simulink model "full"  (Simulink 8.3)
settings: Solver=ode3  StartTime=0.0  StopTime=stop_time  FixedStep=step  RelTol=1e-3
values from neighbouring files (symbols this model uses):
  i_p = i_p_data(i)    [test_2.m]
  J_sum = J_d + 0.2*J_d + J_m/i_p^2    (= 0.011)    [test_2.m]
  K_a = 10/alpha_max    (= 1.5888147442)    [test_2.m]
  k_d = 1/R    (= 3.33333333333)    [test_2.m]
  k_e = U_n/w_0    (= 0.400454372941)    [test_2.m]
  K_I = 10/I_max    (= 0.108225108225)    [test_2.m]
  k_m = M_n/I_n    (= 0.400555555556)    [test_2.m]
  K_u = 10/U_n    (= 0.192307692308)    [test_2.m]
  K_w = 10/w_0    (= 0.0770104563348)    [test_2.m]
  k_y = U_n/U_m    (= 5.2)    [test_2.m]
  M_cm = 0    [test_2.m]
  T_y = 10*10^(-3)    (= 0.01)    [test_2.m]
  T_ya = 10*10^(-3)    (= 0.01)    [test_2.m]
  U = 5    [test_2.m]
settings Model: Creator=Павел  LastModifiedBy=Павел
settings DataIOCC: SignalLoggingSaveFormat=Dataset
settings DebuggingCC: UnderspecifiedInitializationDetection=Simplified  StateNameClashWarn=none
settings GRTTargetCC: CombineOutputUpdateFcns=on  GRTInterface=off

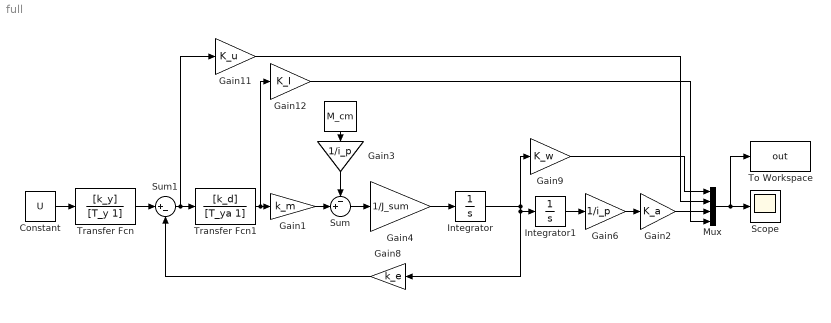
== system full ==
  " " : Constant  Value=M_cm
  Constant : Constant  Value=U
  Gain1 : Gain  Gain=k_m
  Gain11 : Gain  Gain=K_u
  Gain12 : Gain  Gain=K_I
  Gain2 : Gain  Gain=K_a
  Gain3 : Gain  Gain=1/i_p
  Gain4 : Gain  Gain=1/J_sum
  Gain6 : Gain  Gain=1/i_p
  Gain8 : Gain  Gain=k_e
  Gain9 : Gain  Gain=K_w
  Integrator : Integrator
  Integrator1 : Integrator
  Mux : Mux
  Scope : Scope
      settings: TimeRange=0.025712143928036  YMin=0.7292025862068964  YMax=0.7738146551724137
  Sum : Sum  Inputs=-+|
  Sum1 : Sum  Inputs=|+-
  To Workspace : ToWorkspace  VariableName=out  SaveFormat=Structure With Time  SampleTime=-1
  Transfer Fcn : TransferFcn  Numerator=[k_y]  Denominator=[T_y 1]
  Transfer Fcn1 : TransferFcn  Numerator=[k_d]  Denominator=[T_ya 1]
  wires:
  Sum1/1 -> Gain11/1, Transfer Fcn1/1
  Transfer Fcn/1 -> Sum1/1
  Constant/1 -> Transfer Fcn/1
  Gain1/1 -> Sum/2
  Gain3/1 -> Sum/1
  Sum/1 -> Gain4/1
  Gain4/1 -> Integrator/1
  Integrator/1 -> Gain9/1, Integrator1/1, Gain8/1
  Gain8/1 -> Sum1/2
  " "/1 -> Gain3/1
  Mux/1 -> Scope/1, To Workspace/1
  Transfer Fcn1/1 -> Gain12/1, Gain1/1
  Gain9/1 -> Mux/1
  Gain2/1 -> Mux/3
  Gain6/1 -> Gain2/1
  Integrator1/1 -> Gain6/1
  Gain11/1 -> Mux/2
  Gain12/1 -> Mux/4
